simulink model "axis_packet_generator"  (R2020a)
settings: Solver=FixedStepDiscrete  StartTime=0.0  StopTime=inf  RelTol=1e-3
InitFcn:
  | f_system = 256e6;
libraries: hdlsllib x18, simulink x4
settings Model: DataTypeOverride=Off  Creator=david  LastModifiedBy=david
settings OptimizationCC: BlockReduction=off  ConditionallyExecuteInputs=off  DefaultParameterBehavior=Inlined
settings DebuggingCC: AlgebraicLoopMsg=error  SingleTaskRateTransMsg=error
settings HardwareCC: ProdBitPerPointer=32  ProdBitPerSizeT=32  ProdBitPerPtrDiffT=32  ProdLargestAtomicFloat=None  ProdIntDivRoundTo=Undefined  ProdEndianess=Unspecified  ProdWordSize=32  ProdHWDeviceType=ASIC/FPGA->ASIC/FPGA  TargetBitPerPointer=64  TargetBitPerSizeT=64  TargetBitPerPtrDiffT=64  TargetLongLongMode=on  TargetIntDivRoundTo=Zero  TargetEndianess=LittleEndian  TargetWordSize=64  TargetHWDeviceType=Custom Processor->MATLAB Host Computer  ProdEqTarget=off

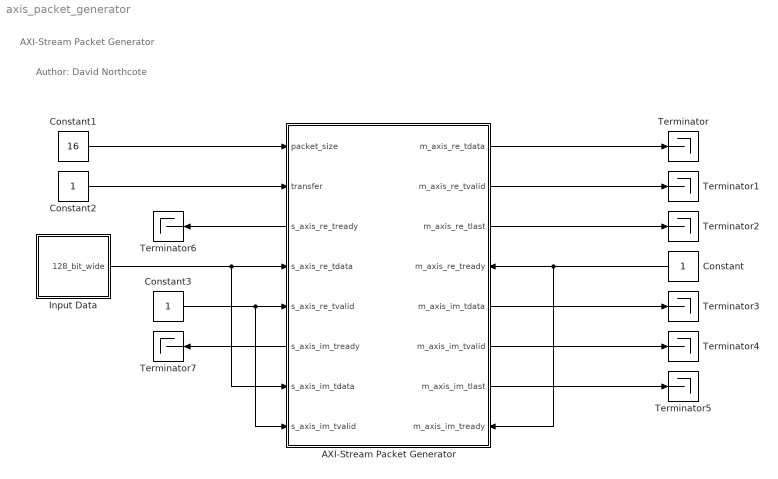
== system axis_packet_generator ==
  note: Author: David Northcote
  note: AXI-Stream Packet Generator
  AXI-Stream Packet Generator : Subsystem  TreatAsAtomicUnit=on
      settings: PortSchema="{\"entries\":[{\"content\":{\"sides\":[{\"content\":{\"connectorIds\":[\"In1\",\"In2\",\"Out7\",\"In3\",\"In4\",\"Out8\",\"In5\",\"In6\"]},\"type\":\"ConnectorPlacement.EquallySpacedRectSide\",\"uuid\":\"239a9995-0b8c-494e-a673-86dd79e3ecbc\"},{\"content\":{\"connectorIds\":[\"Out1\",\"Out2\",\"Out3\",\"In7\",\"Out4\",\"Out5\",\"Out6\",\"In8\"],\"side\":\"RIGHT\"},\"type\":\"ConnectorPlacement.EquallySpacedRectSide\",\"uuid\":\"2e32a57b-a30e-49d7-a7e9-0e4be6c7949e\"},{\"content\":{\"connectorIds\":[],\"side\":\"TOP\"},\"type\":\"ConnectorPlacement.EquallySpacedRectSide\",\"uuid\":\"0fe3c5fd-6b2b-4864-8f33-4697d91e188d\"}]},\"type\":\"ConnectorPlacement.EquallySpacedConnector\",\"uuid\":\"659fe604-1a06-443f-bb23-1784571a6596\"}],\"packageUris\":[\"http://schema.mathworks.com/mf0/Connector/19700101\"],\"version\":\"1.0\"}"
  Constant : Constant  OutDataTypeStr=boolean  SampleTime=-1
  Constant1 : Constant  Value=16  OutDataTypeStr=uint32  SampleTime=-1
  Constant2 : Constant  OutDataTypeStr=uint32  SampleTime=-1
  Constant3 : Constant  OutDataTypeStr=boolean  SampleTime=-1
  Input Data : Subsystem
  Terminator{,1..7} (8 alike) : Terminator
  wires:
  AXI-Stream Packet Generator/1(m_axis_re_tdata) -> Terminator/1
  AXI-Stream Packet Generator/2(m_axis_re_tvalid) -> Terminator1/1
  AXI-Stream Packet Generator/3(m_axis_re_tlast) -> Terminator2/1
  Constant/1 -> AXI-Stream Packet Generator/8(m_axis_im_tready), AXI-Stream Packet Generator/7(m_axis_re_tready)
  AXI-Stream Packet Generator/6(m_axis_im_tlast) -> Terminator5/1
  AXI-Stream Packet Generator/5(m_axis_im_tvalid) -> Terminator4/1
  AXI-Stream Packet Generator/4(m_axis_im_tdata) -> Terminator3/1
  Constant1/1 -> AXI-Stream Packet Generator/1(packet_size)
  AXI-Stream Packet Generator/7(s_axis_re_tready) -> Terminator6/1
  AXI-Stream Packet Generator/8(s_axis_im_tready) -> Terminator7/1
  Constant2/1 -> AXI-Stream Packet Generator/2(transfer)
  Input Data/1(128_bit_wide) -> AXI-Stream Packet Generator/5(s_axis_im_tdata), AXI-Stream Packet Generator/3(s_axis_re_tdata)
  Constant3/1 -> AXI-Stream Packet Generator/6(s_axis_im_tvalid), AXI-Stream Packet Generator/4(s_axis_re_tvalid)

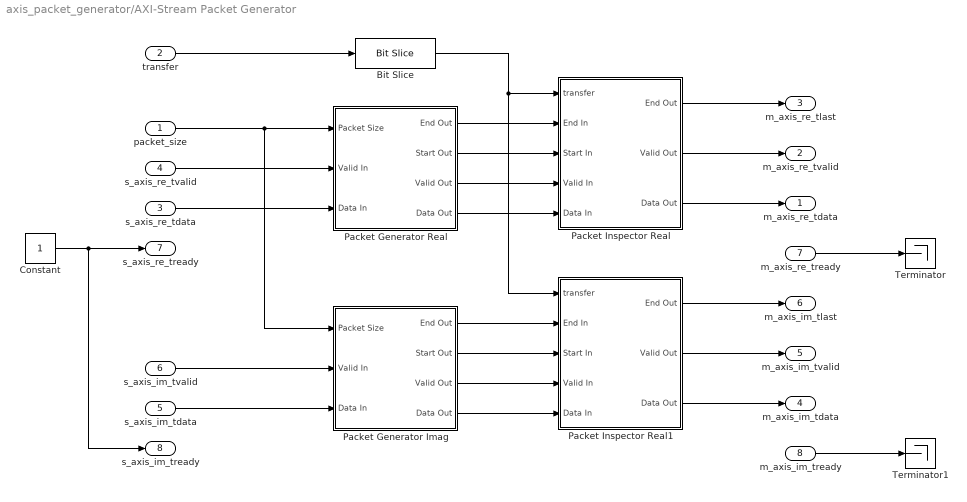
== system axis_packet_generator/AXI-Stream Packet Generator ==
  packet_size : Inport
  transfer : Inport  Port=2
  s_axis_re_tdata : Inport  Port=3
  s_axis_re_tvalid : Inport  Port=4
  s_axis_im_tdata : Inport  Port=5
  s_axis_im_tvalid : Inport  Port=6
  m_axis_re_tready : Inport  Port=7
  m_axis_im_tready : Inport  Port=8
  Bit Slice : hdlsllib/Logic and Bit Operations/Bit Slice  lidx=0  ridx=0
      settings: SourceProductBaseCode=SL
  Constant : Constant  OutDataTypeStr=boolean  SampleTime=-1
  Packet Generator Imag : Subsystem
  Packet Generator Real : Subsystem
  Packet Inspector Real : Subsystem
  Packet Inspector Real1 : Subsystem
  Terminator : Terminator
  Terminator1 : Terminator
  m_axis_re_tdata : Outport
  m_axis_re_tvalid : Outport  Port=2
  m_axis_re_tlast : Outport  Port=3
  m_axis_im_tdata : Outport  Port=4
  m_axis_im_tvalid : Outport  Port=5
  m_axis_im_tlast : Outport  Port=6
  s_axis_re_tready : Outport  Port=7
  s_axis_im_tready : Outport  Port=8
  wires:
  packet_size/1 -> Packet Generator Real/1(Packet Size), Packet Generator Imag/1(Packet Size)
  s_axis_re_tvalid/1 -> Packet Generator Real/2(Valid In)
  s_axis_re_tdata/1 -> Packet Generator Real/3(Data In)
  s_axis_im_tdata/1 -> Packet Generator Imag/3(Data In)
  s_axis_im_tvalid/1 -> Packet Generator Imag/2(Valid In)
  Constant/1 -> s_axis_re_tready/1, s_axis_im_tready/1
  Packet Generator Imag/3(Valid Out) -> Packet Inspector Real1/4(Valid In)
  Packet Generator Imag/4(Data Out) -> Packet Inspector Real1/5(Data In)
  Packet Generator Imag/2(Start Out) -> Packet Inspector Real1/3(Start In)
  Packet Generator Imag/1(End Out) -> Packet Inspector Real1/2(End In)
  transfer/1 -> Bit Slice/1
  Packet Generator Real/1(End Out) -> Packet Inspector Real/2(End In)
  Packet Generator Real/2(Start Out) -> Packet Inspector Real/3(Start In)
  Packet Generator Real/3(Valid Out) -> Packet Inspector Real/4(Valid In)
  Packet Generator Real/4(Data Out) -> Packet Inspector Real/5(Data In)
  Packet Inspector Real/3(Data Out) -> m_axis_re_tdata/1
  Packet Inspector Real/1(End Out) -> m_axis_re_tlast/1
  Packet Inspector Real/2(Valid Out) -> m_axis_re_tvalid/1
  m_axis_re_tready/1 -> Terminator/1
  Packet Inspector Real1/3(Data Out) -> m_axis_im_tdata/1
  Packet Inspector Real1/2(Valid Out) -> m_axis_im_tvalid/1
  Packet Inspector Real1/1(End Out) -> m_axis_im_tlast/1
  m_axis_im_tready/1 -> Terminator1/1
  Bit Slice/1 -> Packet Inspector Real1/1(transfer), Packet Inspector Real/1(transfer)

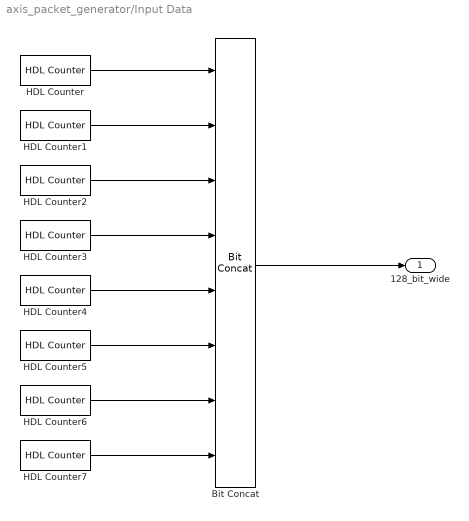
== system axis_packet_generator/Input Data ==
  Bit Concat : hdlsllib/Logic and Bit Operations/Bit Concat  numInputs=8
  HDL Counter : hdlsllib/Sources/HDL Counter  CountType=Free running  CountInit=7  CountStep=8  CountMax=25  CountFromType=Initial value  CountFrom=7  CountResetPort=off  CountLoadPort=off  CountEnbPort=off  CountDirPort=off  CountDataType=Unsigned  CountWordLen=16  CountFracLen=0  CountSampTime=1/f_system
  HDL Counter1 : hdlsllib/Sources/HDL Counter  CountType=Free running  CountInit=6  CountStep=8  CountMax=25  CountFromType=Initial value  CountFrom=6  CountResetPort=off  CountLoadPort=off  CountEnbPort=off  CountDirPort=off  CountDataType=Unsigned  CountWordLen=16  CountFracLen=0  CountSampTime=1/f_system
  HDL Counter2 : hdlsllib/Sources/HDL Counter  CountType=Free running  CountInit=5  CountStep=8  CountMax=25  CountFromType=Initial value  CountFrom=5  CountResetPort=off  CountLoadPort=off  CountEnbPort=off  CountDirPort=off  CountDataType=Unsigned  CountWordLen=16  CountFracLen=0  CountSampTime=1/f_system
  HDL Counter3 : hdlsllib/Sources/HDL Counter  CountType=Free running  CountInit=4  CountStep=8  CountMax=25  CountFromType=Initial value  CountFrom=4  CountResetPort=off  CountLoadPort=off  CountEnbPort=off  CountDirPort=off  CountDataType=Unsigned  CountWordLen=16  CountFracLen=0  CountSampTime=1/f_system
  HDL Counter4 : hdlsllib/Sources/HDL Counter  CountType=Free running  CountInit=3  CountStep=8  CountMax=25  CountFromType=Initial value  CountFrom=3  CountResetPort=off  CountLoadPort=off  CountEnbPort=off  CountDirPort=off  CountDataType=Unsigned  CountWordLen=16  CountFracLen=0  CountSampTime=1/f_system
  HDL Counter5 : hdlsllib/Sources/HDL Counter  CountType=Free running  CountInit=2  CountStep=8  CountMax=25  CountFromType=Initial value  CountFrom=2  CountResetPort=off  CountLoadPort=off  CountEnbPort=off  CountDirPort=off  CountDataType=Unsigned  CountWordLen=16  CountFracLen=0  CountSampTime=1/f_system
  HDL Counter6 : hdlsllib/Sources/HDL Counter  CountType=Free running  CountInit=1  CountStep=8  CountMax=25  CountFromType=Initial value  CountFrom=1  CountResetPort=off  CountLoadPort=off  CountEnbPort=off  CountDirPort=off  CountDataType=Unsigned  CountWordLen=16  CountFracLen=0  CountSampTime=1/f_system
  HDL Counter7 : hdlsllib/Sources/HDL Counter  CountType=Free running  CountInit=0  CountStep=8  CountMax=25  CountFromType=Initial value  CountFrom=0  CountResetPort=off  CountLoadPort=off  CountEnbPort=off  CountDirPort=off  CountDataType=Unsigned  CountWordLen=16  CountFracLen=0  CountSampTime=1/f_system
  128_bit_wide : Outport
  wires:
  HDL Counter7/1 -> Bit Concat/8
  HDL Counter2/1 -> Bit Concat/3
  HDL Counter4/1 -> Bit Concat/5
  HDL Counter6/1 -> Bit Concat/7
  HDL Counter3/1 -> Bit Concat/4
  HDL Counter1/1 -> Bit Concat/2
  HDL Counter/1 -> Bit Concat/1
  HDL Counter5/1 -> Bit Concat/6
  Bit Concat/1 -> 128_bit_wide/1

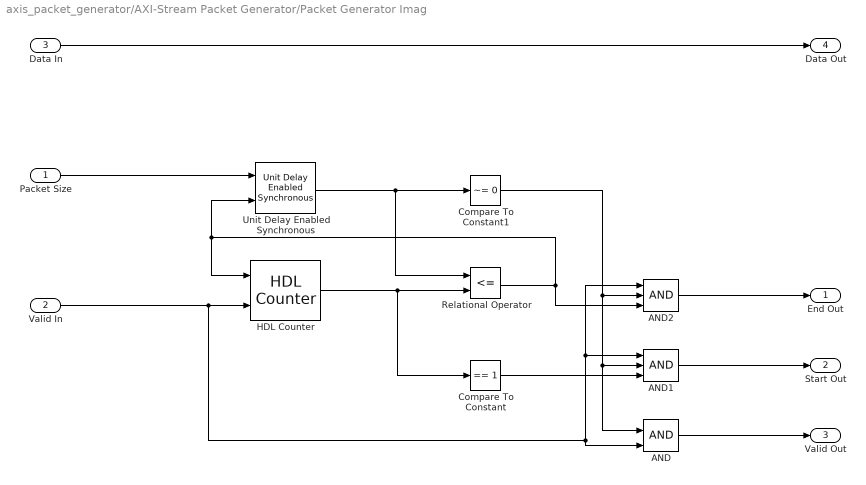
== system axis_packet_generator/AXI-Stream Packet Generator/Packet Generator Imag ==
  Packet Size : Inport
  Valid In : Inport  Port=2
  Data In : Inport  Port=3
  AND : Logic  IconShape=distinctive  AllPortsSameDT=off  OutDataTypeStr=boolean
  AND1 : Logic  Inputs=3  IconShape=distinctive  AllPortsSameDT=off  OutDataTypeStr=boolean
  AND2 : Logic  Inputs=3  IconShape=distinctive  AllPortsSameDT=off  OutDataTypeStr=boolean
  Compare To Constant : simulink/Logic and Bit Operations/Compare To Constant  relop===  const=1  OutDataTypeStr=boolean
  Compare To Constant1 : simulink/Logic and Bit Operations/Compare To Constant  relop=~=  const=0  OutDataTypeStr=boolean
  HDL Counter : hdlsllib/Sources/HDL Counter  CountType=Free running  CountInit=1  CountStep=1  CountMax=25  CountFromType=Initial value  CountFrom=1  CountResetPort=on  CountLoadPort=off  CountEnbPort=on  CountDirPort=off  CountDataType=Unsigned  CountWordLen=32  CountFracLen=0  CountSampTime=1
  Relational Operator : RelationalOperator  Operator=<=  OutDataTypeStr=boolean  RndMeth=Simplest
  Unit Delay Enabled Synchronous : hdlsllib/Discrete/Unit Delay Enabled Synchronous  InitialCondition=0.0  SampleTime=-1
      settings: SourceProductBaseCode=SL
  End Out : Outport
  Start Out : Outport  Port=2
  Valid Out : Outport  Port=3
  Data Out : Outport  Port=4
  wires:
  Data In/1 -> Data Out/1
  AND2/1 -> End Out/1
  AND/1 -> Valid Out/1
  AND1/1 -> Start Out/1
  Compare To Constant/1 -> AND1/3
  Relational Operator/1 -> AND2/3, Unit Delay Enabled Synchronous/2, HDL Counter/1
  Packet Size/1 -> Unit Delay Enabled Synchronous/1
  Compare To Constant1/1 -> AND/1, AND1/2, AND2/2
  HDL Counter/1 -> Compare To Constant/1, Relational Operator/2
  Valid In/1 -> HDL Counter/2, AND/2, AND1/1, AND2/1
  Unit Delay Enabled Synchronous/1 -> Relational Operator/1, Compare To Constant1/1

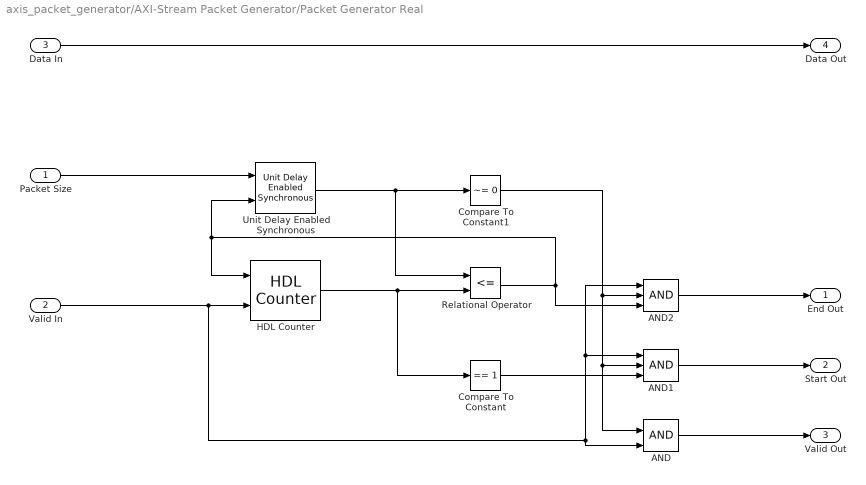
== system axis_packet_generator/AXI-Stream Packet Generator/Packet Generator Real ==
  Packet Size : Inport
  Valid In : Inport  Port=2
  Data In : Inport  Port=3
  AND : Logic  IconShape=distinctive  AllPortsSameDT=off  OutDataTypeStr=boolean
  AND1 : Logic  Inputs=3  IconShape=distinctive  AllPortsSameDT=off  OutDataTypeStr=boolean
  AND2 : Logic  Inputs=3  IconShape=distinctive  AllPortsSameDT=off  OutDataTypeStr=boolean
  Compare To Constant : simulink/Logic and Bit Operations/Compare To Constant  relop===  const=1  OutDataTypeStr=boolean
  Compare To Constant1 : simulink/Logic and Bit Operations/Compare To Constant  relop=~=  const=0  OutDataTypeStr=boolean
  HDL Counter : hdlsllib/Sources/HDL Counter  CountType=Free running  CountInit=1  CountStep=1  CountMax=25  CountFromType=Initial value  CountFrom=1  CountResetPort=on  CountLoadPort=off  CountEnbPort=on  CountDirPort=off  CountDataType=Unsigned  CountWordLen=32  CountFracLen=0  CountSampTime=1
  Relational Operator : RelationalOperator  Operator=<=  OutDataTypeStr=boolean  RndMeth=Simplest
  Unit Delay Enabled Synchronous : hdlsllib/Discrete/Unit Delay Enabled Synchronous  InitialCondition=0.0  SampleTime=-1
      settings: SourceProductBaseCode=SL
  End Out : Outport
  Start Out : Outport  Port=2
  Valid Out : Outport  Port=3
  Data Out : Outport  Port=4
  wires:
  Unit Delay Enabled Synchronous/1 -> Compare To Constant1/1, Relational Operator/1
  Valid In/1 -> AND2/1, AND1/1, AND/2, HDL Counter/2
  HDL Counter/1 -> Relational Operator/2, Compare To Constant/1
  Compare To Constant1/1 -> AND2/2, AND1/2, AND/1
  Packet Size/1 -> Unit Delay Enabled Synchronous/1
  Relational Operator/1 -> HDL Counter/1, Unit Delay Enabled Synchronous/2, AND2/3
  Compare To Constant/1 -> AND1/3
  AND1/1 -> Start Out/1
  AND/1 -> Valid Out/1
  AND2/1 -> End Out/1
  Data In/1 -> Data Out/1

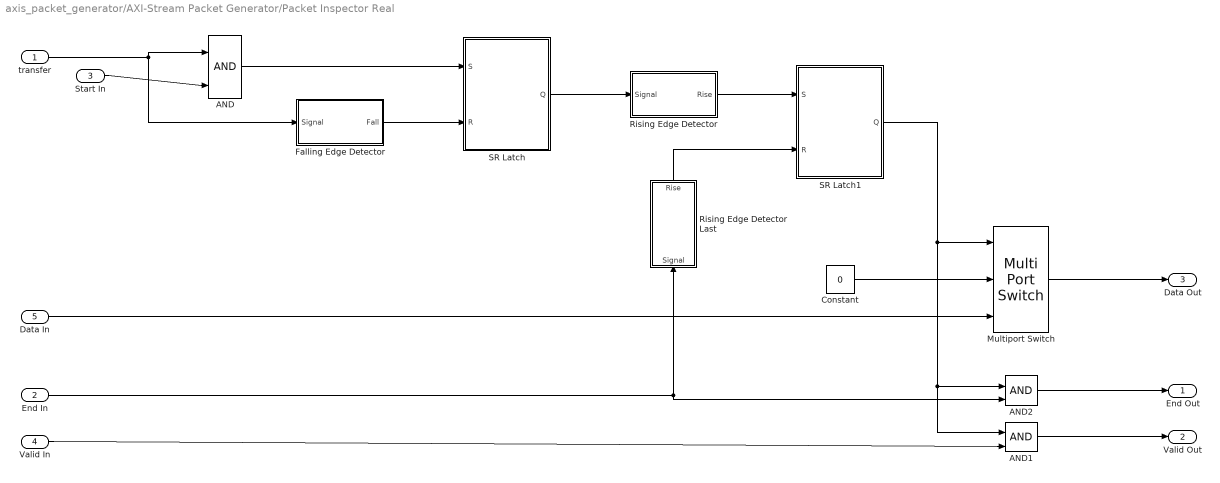
== system axis_packet_generator/AXI-Stream Packet Generator/Packet Inspector Real ==
  transfer : Inport
  End In : Inport  Port=2
  Start In : Inport  Port=3
  Valid In : Inport  Port=4
  Data In : Inport  Port=5
  AND : Logic  IconShape=distinctive  AllPortsSameDT=off  OutDataTypeStr=boolean
  AND1 : Logic  IconShape=distinctive  AllPortsSameDT=off  OutDataTypeStr=boolean
  AND2 : Logic  IconShape=distinctive  AllPortsSameDT=off  OutDataTypeStr=boolean
  Constant : Constant  Value=0  OutDataTypeStr=Inherit: Inherit via back propagation  SampleTime=-1
  Falling Edge Detector : Subsystem
  Multiport Switch : MultiPortSwitch  DataPortOrder=Zero-based contiguous  Inputs=2  zeroidx=on
  Rising Edge Detector Last : Subsystem
  Rising Edge Detector : Subsystem
  SR Latch : Subsystem
  SR Latch1 : Subsystem
  End Out : Outport
  Valid Out : Outport  Port=2
  Data Out : Outport  Port=3
  wires:
  transfer/1 -> AND/1, Falling Edge Detector/1(Signal)
  Start In/1 -> AND/2
  AND/1 -> SR Latch/1(S)
  Falling Edge Detector/1(Fall) -> SR Latch/2(R)
  SR Latch/1(Q) -> Rising Edge Detector/1(Signal)
  Rising Edge Detector/1(Rise) -> SR Latch1/1(S)
  Rising Edge Detector Last/1(Rise) -> SR Latch1/2(R)
  SR Latch1/1(Q) -> AND2/1, AND1/1, Multiport Switch/1
  Constant/1 -> Multiport Switch/2
  Data In/1 -> Multiport Switch/3
  Valid In/1 -> AND1/2
  End In/1 -> Rising Edge Detector Last/1(Signal), AND2/2
  AND1/1 -> Valid Out/1
  Multiport Switch/1 -> Data Out/1
  AND2/1 -> End Out/1

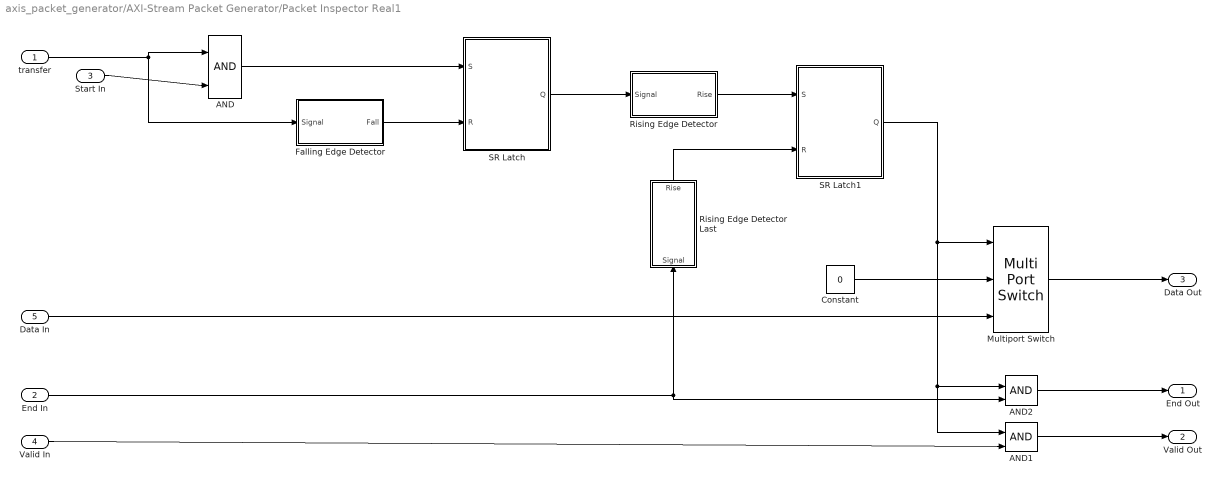
== system axis_packet_generator/AXI-Stream Packet Generator/Packet Inspector Real1 ==
  transfer : Inport
  End In : Inport  Port=2
  Start In : Inport  Port=3
  Valid In : Inport  Port=4
  Data In : Inport  Port=5
  AND : Logic  IconShape=distinctive  AllPortsSameDT=off  OutDataTypeStr=boolean
  AND1 : Logic  IconShape=distinctive  AllPortsSameDT=off  OutDataTypeStr=boolean
  AND2 : Logic  IconShape=distinctive  AllPortsSameDT=off  OutDataTypeStr=boolean
  Constant : Constant  Value=0  OutDataTypeStr=Inherit: Inherit via back propagation  SampleTime=-1
  Falling Edge Detector : Subsystem
  Multiport Switch : MultiPortSwitch  DataPortOrder=Zero-based contiguous  Inputs=2  zeroidx=on
  Rising Edge Detector Last : Subsystem
  Rising Edge Detector : Subsystem
  SR Latch : Subsystem
  SR Latch1 : Subsystem
  End Out : Outport
  Valid Out : Outport  Port=2
  Data Out : Outport  Port=3
  wires:
  AND2/1 -> End Out/1
  Multiport Switch/1 -> Data Out/1
  AND1/1 -> Valid Out/1
  End In/1 -> AND2/2, Rising Edge Detector Last/1(Signal)
  Valid In/1 -> AND1/2
  Data In/1 -> Multiport Switch/3
  Constant/1 -> Multiport Switch/2
  SR Latch1/1(Q) -> Multiport Switch/1, AND1/1, AND2/1
  Rising Edge Detector Last/1(Rise) -> SR Latch1/2(R)
  Rising Edge Detector/1(Rise) -> SR Latch1/1(S)
  SR Latch/1(Q) -> Rising Edge Detector/1(Signal)
  Falling Edge Detector/1(Fall) -> SR Latch/2(R)
  AND/1 -> SR Latch/1(S)
  Start In/1 -> AND/2
  transfer/1 -> Falling Edge Detector/1(Signal), AND/1

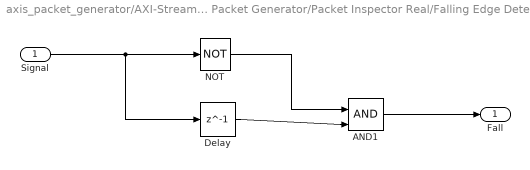
== system axis_packet_generator/AXI-Stream Packet Generator/Packet Inspector Real/Falling Edge Detector ==
  Signal : Inport
  AND1 : Logic  IconShape=distinctive  AllPortsSameDT=off  OutDataTypeStr=boolean
  Delay : Delay  DelayLength=1
  NOT : Logic  Operator=NOT  IconShape=distinctive  AllPortsSameDT=off  OutDataTypeStr=boolean
  Fall : Outport
  wires:
  Delay/1 -> AND1/2
  Signal/1 -> NOT/1, Delay/1
  AND1/1 -> Fall/1
  NOT/1 -> AND1/1

== system axis_packet_generator/AXI-Stream Packet Generator/Packet Inspector Real/Rising Edge Detector Last ==
  Signal : Inport
  AND1 : Logic  IconShape=distinctive  AllPortsSameDT=off  OutDataTypeStr=boolean
  Delay : Delay  DelayLength=1
  NOT : Logic  Operator=NOT  IconShape=distinctive  AllPortsSameDT=off  OutDataTypeStr=boolean
  Rise : Outport
  wires:
  NOT/1 -> Delay/1
  Delay/1 -> AND1/2
  Signal/1 -> NOT/1, AND1/1
  AND1/1 -> Rise/1

== system axis_packet_generator/AXI-Stream Packet Generator/Packet Inspector Real/Rising Edge Detector ==
  Signal : Inport
  AND1 : Logic  IconShape=distinctive  AllPortsSameDT=off  OutDataTypeStr=boolean
  Delay : Delay  DelayLength=1
  NOT : Logic  Operator=NOT  IconShape=distinctive  AllPortsSameDT=off  OutDataTypeStr=boolean
  Rise : Outport
  wires:
  AND1/1 -> Rise/1
  Signal/1 -> AND1/1, NOT/1
  Delay/1 -> AND1/2
  NOT/1 -> Delay/1

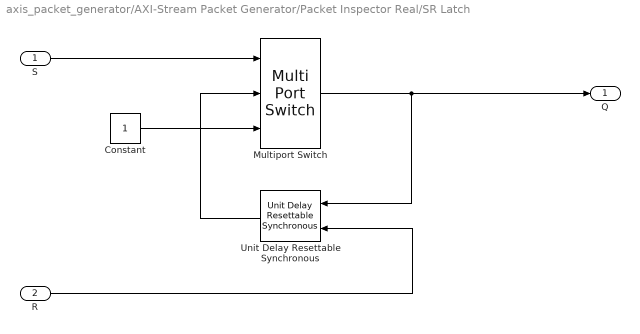
== system axis_packet_generator/AXI-Stream Packet Generator/Packet Inspector Real/SR Latch ==
  S : Inport
  R : Inport  Port=2
  Constant : Constant  OutDataTypeStr=boolean  SampleTime=-1
  Multiport Switch : MultiPortSwitch  DataPortOrder=Zero-based contiguous  Inputs=2  zeroidx=on
  Unit Delay Resettable Synchronous : hdlsllib/Discrete/Unit Delay Resettable Synchronous  InitialCondition=0.0  SampleTime=-1
      settings: SourceProductBaseCode=SL
  Q : Outport
  wires:
  R/1 -> Unit Delay Resettable Synchronous/2
  Multiport Switch/1 -> Q/1, Unit Delay Resettable Synchronous/1
  Constant/1 -> Multiport Switch/3
  Unit Delay Resettable Synchronous/1 -> Multiport Switch/2
  S/1 -> Multiport Switch/1

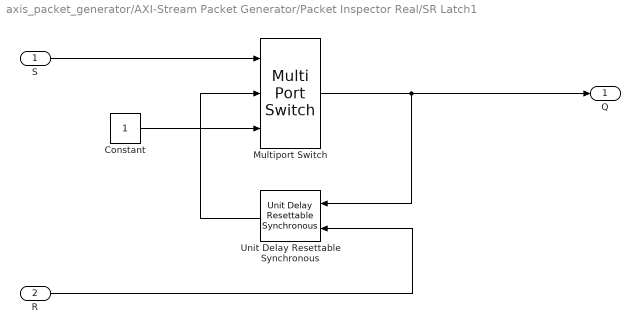
== system axis_packet_generator/AXI-Stream Packet Generator/Packet Inspector Real/SR Latch1 ==
  S : Inport
  R : Inport  Port=2
  Constant : Constant  OutDataTypeStr=boolean  SampleTime=-1
  Multiport Switch : MultiPortSwitch  DataPortOrder=Zero-based contiguous  Inputs=2  zeroidx=on
  Unit Delay Resettable Synchronous : hdlsllib/Discrete/Unit Delay Resettable Synchronous  InitialCondition=0.0  SampleTime=-1
      settings: SourceProductBaseCode=SL
  Q : Outport
  wires:
  S/1 -> Multiport Switch/1
  Unit Delay Resettable Synchronous/1 -> Multiport Switch/2
  Constant/1 -> Multiport Switch/3
  Multiport Switch/1 -> Unit Delay Resettable Synchronous/1, Q/1
  R/1 -> Unit Delay Resettable Synchronous/2

== system axis_packet_generator/AXI-Stream Packet Generator/Packet Inspector Real1/Falling Edge Detector ==
  Signal : Inport
  AND1 : Logic  IconShape=distinctive  AllPortsSameDT=off  OutDataTypeStr=boolean
  Delay : Delay  DelayLength=1
  NOT : Logic  Operator=NOT  IconShape=distinctive  AllPortsSameDT=off  OutDataTypeStr=boolean
  Fall : Outport
  wires:
  NOT/1 -> AND1/1
  AND1/1 -> Fall/1
  Signal/1 -> Delay/1, NOT/1
  Delay/1 -> AND1/2

== system axis_packet_generator/AXI-Stream Packet Generator/Packet Inspector Real1/Rising Edge Detector Last ==
  Signal : Inport
  AND1 : Logic  IconShape=distinctive  AllPortsSameDT=off  OutDataTypeStr=boolean
  Delay : Delay  DelayLength=1
  NOT : Logic  Operator=NOT  IconShape=distinctive  AllPortsSameDT=off  OutDataTypeStr=boolean
  Rise : Outport
  wires:
  AND1/1 -> Rise/1
  Signal/1 -> AND1/1, NOT/1
  Delay/1 -> AND1/2
  NOT/1 -> Delay/1

== system axis_packet_generator/AXI-Stream Packet Generator/Packet Inspector Real1/Rising Edge Detector ==
  Signal : Inport
  AND1 : Logic  IconShape=distinctive  AllPortsSameDT=off  OutDataTypeStr=boolean
  Delay : Delay  DelayLength=1
  NOT : Logic  Operator=NOT  IconShape=distinctive  AllPortsSameDT=off  OutDataTypeStr=boolean
  Rise : Outport
  wires:
  NOT/1 -> Delay/1
  Delay/1 -> AND1/2
  Signal/1 -> NOT/1, AND1/1
  AND1/1 -> Rise/1

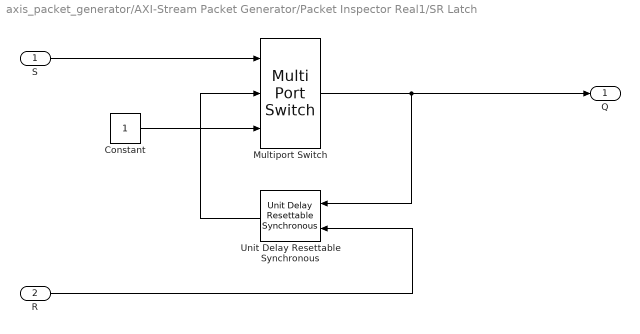
== system axis_packet_generator/AXI-Stream Packet Generator/Packet Inspector Real1/SR Latch ==
  S : Inport
  R : Inport  Port=2
  Constant : Constant  OutDataTypeStr=boolean  SampleTime=-1
  Multiport Switch : MultiPortSwitch  DataPortOrder=Zero-based contiguous  Inputs=2  zeroidx=on
  Unit Delay Resettable Synchronous : hdlsllib/Discrete/Unit Delay Resettable Synchronous  InitialCondition=0.0  SampleTime=-1
      settings: SourceProductBaseCode=SL
  Q : Outport
  wires:
  S/1 -> Multiport Switch/1
  Unit Delay Resettable Synchronous/1 -> Multiport Switch/2
  Constant/1 -> Multiport Switch/3
  Multiport Switch/1 -> Unit Delay Resettable Synchronous/1, Q/1
  R/1 -> Unit Delay Resettable Synchronous/2

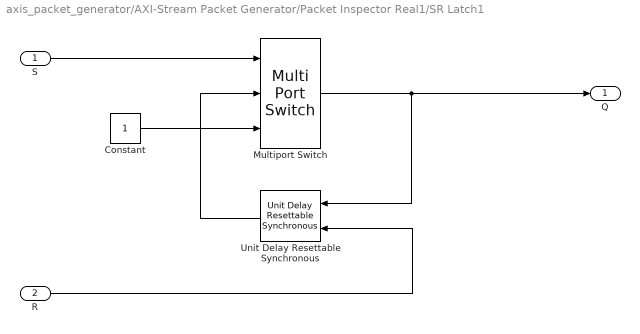
== system axis_packet_generator/AXI-Stream Packet Generator/Packet Inspector Real1/SR Latch1 ==
  S : Inport
  R : Inport  Port=2
  Constant : Constant  OutDataTypeStr=boolean  SampleTime=-1
  Multiport Switch : MultiPortSwitch  DataPortOrder=Zero-based contiguous  Inputs=2  zeroidx=on
  Unit Delay Resettable Synchronous : hdlsllib/Discrete/Unit Delay Resettable Synchronous  InitialCondition=0.0  SampleTime=-1
      settings: SourceProductBaseCode=SL
  Q : Outport
  wires:
  R/1 -> Unit Delay Resettable Synchronous/2
  Multiport Switch/1 -> Q/1, Unit Delay Resettable Synchronous/1
  Constant/1 -> Multiport Switch/3
  Unit Delay Resettable Synchronous/1 -> Multiport Switch/2
  S/1 -> Multiport Switch/1
